simulink model "basis2"  (Simulink 6.6)
settings: Solver=ode45  StartTime=0.0  StopTime=5000  RelTol=1e-3
libraries: simulink x35, dspstat3 x3
settings Model: Creator=Paul.Dourbal  LastModifiedBy=Paul.Dourbal

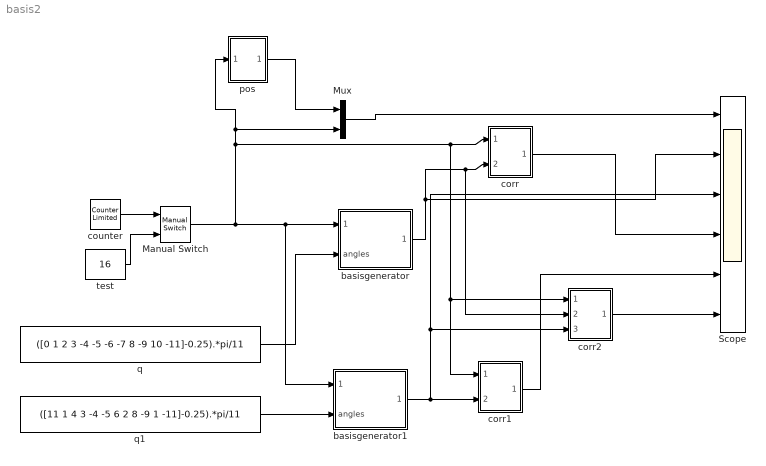
== system basis2 ==
  Manual Switch : simulink/Signal Routing/Manual Switch  SystemSampleTime=-1  sw=1  action=0  varsize=off
  Mux : Mux  Inputs=2
  Scope : Scope  NumInputPorts=6
      settings: TimeRange=64  YMin=-0.15~0~-1~-5~-5~-5  YMax=0.4~65~10~5~5~5
  basisgenerator : Subsystem
  basisgenerator1 : Subsystem
  corr : Subsystem
  corr1 : Subsystem
  corr2 : Subsystem
  counter : simulink/Sources/Counter Limited  SystemSampleTime=-1  uplimit=2^(3+3)-1  tsamp=1
  pos : Subsystem
  q : Constant  Value=([0 1 2 3 -4 -5 -6 -7 8 -9 10 -11]-0.25).*pi/11
  q1 : Constant  Value=([11 1 4 3 -4 -5 6 2 8 -9 1 -11]-0.25).*pi/11
  test : Constant  Value=16  OutDataTypeMode=uint8
  wires:
  basisgenerator/1(samples) -> Scope/2, corr/2(In2), corr2/2(sig1)
  test/1 -> Manual Switch/2
  counter/1 -> Manual Switch/1
  Manual Switch/1 -> pos/1(In1), Mux/2, corr/1(In1), corr1/1(In1), corr2/1(index), basisgenerator/1(counter), basisgenerator1/1(counter)
  pos/1(Out1) -> Mux/1
  Mux/1 -> Scope/1
  q1/1 -> basisgenerator1/2(angles)
  q/1 -> basisgenerator/2(angles)
  basisgenerator1/1(samples) -> corr1/2(In2), Scope/3, corr2/3(sig2)
  corr/1(Out1) -> Scope/4
  corr1/1(Out1) -> Scope/5
  corr2/1(Out1) -> Scope/6

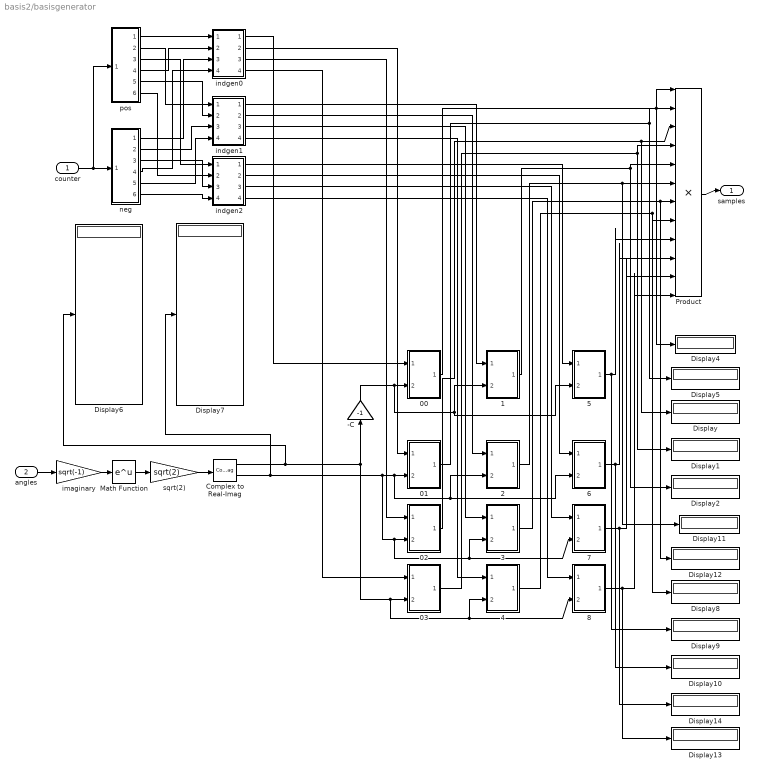
== system basis2/basisgenerator ==
  counter : Inport
  angles : Inport  Port=2
  -C : Gain  Orientation=up  Gain=-1
  00 : Subsystem
  01 : Subsystem
  02 : Subsystem
  03 : Subsystem
  1 : Subsystem
  2 : Subsystem
  3 : Subsystem
  4 : Subsystem
  5 : Subsystem
  6 : Subsystem
  7 : Subsystem
  8 : Subsystem
  Complex to Real-Imag : ComplexToRealImag
  Display{,1..2,4..14} (14 alike) : Display
  Math Function : Math  OutputSignalType=complex  SaturateOnIntegerOverflow=on
  Product : Product  Inputs=12  RndMeth=Zero
  imaginary : Gain  Gain=sqrt(-1)
  indgen0 : Subsystem
  indgen1 : Subsystem
  indgen2 : Subsystem
  neg : Subsystem
  pos : Subsystem
  sqrt(2) : Gain  Gain=sqrt(2)
  samples : Outport
  wires:
  8/1(Out1) -> Product/12, Display13/1
  7/1(Out1) -> Product/11, Display14/1
  6/1(Out1) -> Product/10, Display10/1
  5/1(Out1) -> Product/9, Display9/1
  4/1(Out1) -> Product/8, Display8/1
  3/1(Out1) -> Product/7, Display12/1
  2/1(Out1) -> Product/6, Display11/1
  1/1(Out1) -> Product/5, Display2/1
  03/1(Out1) -> Product/4, Display1/1
  02/1(Out1) -> Product/3, Display/1
  01/1(Out1) -> Product/2, Display5/1
  00/1(Out1) -> Product/1, Display4/1
  indgen2/4(Out4) -> 8/1(In1)
  indgen2/3(Out3) -> 7/1(In1)
  indgen2/2(Out2) -> 6/1(In1)
  indgen2/1(Out1) -> 5/1(In1)
  indgen1/4(Out4) -> 4/1(In1)
  indgen1/3(Out3) -> 3/1(In1)
  indgen1/2(Out2) -> 2/1(In1)
  indgen1/1(Out1) -> 1/1(In1)
  indgen0/4(Out4) -> 03/1(In1)
  indgen0/3(Out3) -> 02/1(In1)
  indgen0/2(Out2) -> 01/1(In1)
  indgen0/1(Out1) -> 00/1(In1)
  -C/1 -> 00/2(In2), 1/2(In2), 5/2(In2)
  neg/6(Out6) -> indgen2/4(In4)
  neg/3(Out3) -> indgen2/3(In3)
  pos/6(Out6) -> indgen2/2(In2)
  pos/3(Out3) -> indgen2/1(In1)
  neg/5(Out5) -> indgen1/4(In4)
  neg/2(Out2) -> indgen1/3(In3)
  pos/5(Out5) -> indgen1/2(In2)
  pos/2(Out2) -> indgen1/1(In1)
  neg/4(Out4) -> indgen0/4(In4)
  neg/1(Out1) -> indgen0/3(In3)
  pos/4(Out4) -> indgen0/2(In2)
  pos/1(Out1) -> indgen0/1(In1)
  Complex to Real-Imag/2 -> 01/2(In2), 2/2(In2), 6/2(In2), 02/2(In2), 3/2(In2), 7/2(In2), Display7/1
  Complex to Real-Imag/1 -> -C/1, 03/2(In2), 4/2(In2), 8/2(In2), Display6/1
  sqrt(2)/1 -> Complex to Real-Imag/1
  Math Function/1 -> sqrt(2)/1
  imaginary/1 -> Math Function/1
  counter/1 -> neg/1(In1), pos/1(In1)
  Product/1 -> samples/1
  angles/1 -> imaginary/1

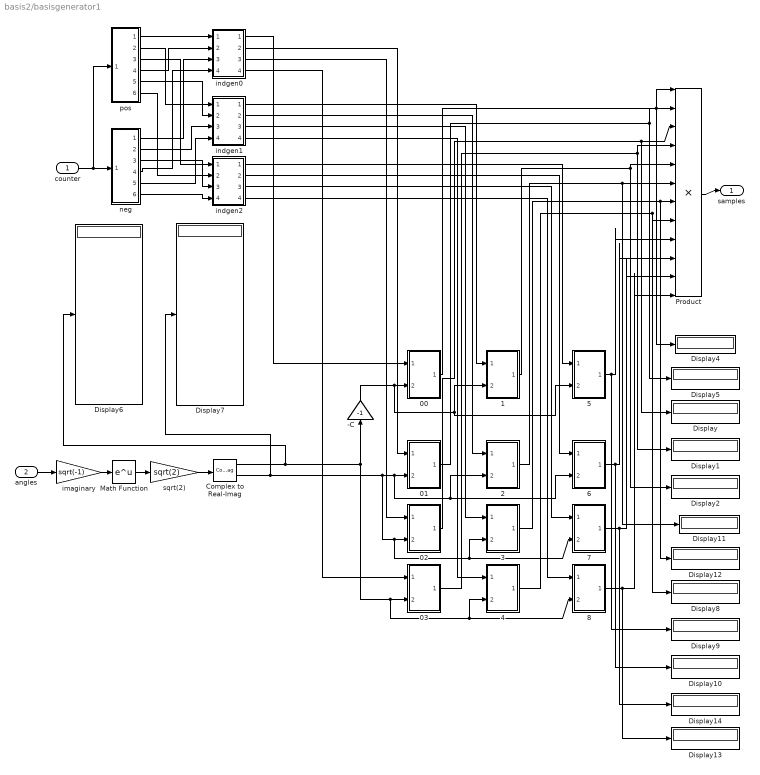
== system basis2/basisgenerator1 ==
  counter : Inport
  angles : Inport  Port=2
  -C : Gain  Orientation=up  Gain=-1
  00 : Subsystem
  01 : Subsystem
  02 : Subsystem
  03 : Subsystem
  1 : Subsystem
  2 : Subsystem
  3 : Subsystem
  4 : Subsystem
  5 : Subsystem
  6 : Subsystem
  7 : Subsystem
  8 : Subsystem
  Complex to Real-Imag : ComplexToRealImag
  Display{,1..2,4..14} (14 alike) : Display
  Math Function : Math  OutputSignalType=complex  SaturateOnIntegerOverflow=on
  Product : Product  Inputs=12  RndMeth=Zero
  imaginary : Gain  Gain=sqrt(-1)
  indgen0 : Subsystem
  indgen1 : Subsystem
  indgen2 : Subsystem
  neg : Subsystem
  pos : Subsystem
  sqrt(2) : Gain  Gain=sqrt(2)
  samples : Outport
  wires:
  8/1(Out1) -> Product/12, Display13/1
  7/1(Out1) -> Product/11, Display14/1
  6/1(Out1) -> Product/10, Display10/1
  5/1(Out1) -> Product/9, Display9/1
  4/1(Out1) -> Product/8, Display8/1
  3/1(Out1) -> Product/7, Display12/1
  2/1(Out1) -> Product/6, Display11/1
  1/1(Out1) -> Product/5, Display2/1
  03/1(Out1) -> Product/4, Display1/1
  02/1(Out1) -> Product/3, Display/1
  01/1(Out1) -> Product/2, Display5/1
  00/1(Out1) -> Product/1, Display4/1
  indgen2/4(Out4) -> 8/1(In1)
  indgen2/3(Out3) -> 7/1(In1)
  indgen2/2(Out2) -> 6/1(In1)
  indgen2/1(Out1) -> 5/1(In1)
  indgen1/4(Out4) -> 4/1(In1)
  indgen1/3(Out3) -> 3/1(In1)
  indgen1/2(Out2) -> 2/1(In1)
  indgen1/1(Out1) -> 1/1(In1)
  indgen0/4(Out4) -> 03/1(In1)
  indgen0/3(Out3) -> 02/1(In1)
  indgen0/2(Out2) -> 01/1(In1)
  indgen0/1(Out1) -> 00/1(In1)
  -C/1 -> 00/2(In2), 1/2(In2), 5/2(In2)
  neg/6(Out6) -> indgen2/4(In4)
  neg/3(Out3) -> indgen2/3(In3)
  pos/6(Out6) -> indgen2/2(In2)
  pos/3(Out3) -> indgen2/1(In1)
  neg/5(Out5) -> indgen1/4(In4)
  neg/2(Out2) -> indgen1/3(In3)
  pos/5(Out5) -> indgen1/2(In2)
  pos/2(Out2) -> indgen1/1(In1)
  neg/4(Out4) -> indgen0/4(In4)
  neg/1(Out1) -> indgen0/3(In3)
  pos/4(Out4) -> indgen0/2(In2)
  pos/1(Out1) -> indgen0/1(In1)
  Complex to Real-Imag/2 -> 01/2(In2), 2/2(In2), 6/2(In2), 02/2(In2), 3/2(In2), 7/2(In2), Display7/1
  Complex to Real-Imag/1 -> -C/1, 03/2(In2), 4/2(In2), 8/2(In2), Display6/1
  sqrt(2)/1 -> Complex to Real-Imag/1
  Math Function/1 -> sqrt(2)/1
  imaginary/1 -> Math Function/1
  counter/1 -> neg/1(In1), pos/1(In1)
  Product/1 -> samples/1
  angles/1 -> imaginary/1

== system basis2/corr ==
  In1 : Inport
  In2 : Inport  Port=2
  Autocorrelation : dspstat3/Autocorrelation  DialogController=dspDDGCreate  DialogControllerArgs=DataTag0  AllPositiveLags=on  maxlag=36  bias=None  domain=Time  roundingMode=Floor  overflowMode=off
  Tapped Delay : simulink/Discrete/Tapped Delay  vinit=0.0  samptime=1/64  NumDelays=64  DelayOrder=Oldest  includeCurrent=off
  mux : Subsystem
  Out1 : Outport
  wires:
  Tapped Delay/1 -> Autocorrelation/1
  Autocorrelation/1 -> mux/2(In2)
  In1/1 -> mux/1(In1)
  In2/1 -> Tapped Delay/1
  mux/1(Out1) -> Out1/1

== system basis2/corr1 ==
  In1 : Inport
  In2 : Inport  Port=2
  Autocorrelation : dspstat3/Autocorrelation  DialogController=dspDDGCreate  DialogControllerArgs=DataTag1  AllPositiveLags=on  maxlag=36  bias=None  domain=Time  roundingMode=Floor  overflowMode=off
  Tapped Delay : simulink/Discrete/Tapped Delay  vinit=0.0  samptime=1/64  NumDelays=64  DelayOrder=Oldest  includeCurrent=off
  mux : Subsystem
  Out1 : Outport
  wires:
  Tapped Delay/1 -> Autocorrelation/1
  Autocorrelation/1 -> mux/2(In2)
  In1/1 -> mux/1(In1)
  In2/1 -> Tapped Delay/1
  mux/1(Out1) -> Out1/1

== system basis2/corr2 ==
  index : Inport
  sig1 : Inport  Port=2
  sig2 : Inport  Port=3
  Correlation : dspstat3/Correlation  DialogController=dspDDGCreate  DialogControllerArgs=DataTag2  domain=Time  roundingMode=Floor  overflowMode=off
  Tapped Delay : simulink/Discrete/Tapped Delay  vinit=0.0  samptime=1/64  NumDelays=64  DelayOrder=Oldest  includeCurrent=off
  Tapped Delay1 : simulink/Discrete/Tapped Delay  vinit=0.0  samptime=1/64  NumDelays=64  DelayOrder=Oldest  includeCurrent=off
  mux : Subsystem
  Out1 : Outport
  wires:
  Tapped Delay/1 -> Correlation/1
  Correlation/1 -> mux/2(In2)
  index/1 -> mux/1(In1)
  sig1/1 -> Tapped Delay/1
  mux/1(Out1) -> Out1/1
  sig2/1 -> Tapped Delay1/1
  Tapped Delay1/1 -> Correlation/2

== system basis2/pos ==
  In1 : Inport  Orientation=up
  Extract Bits3 : simulink/Logic and Bit Operations/Extract Bits  SystemSampleTime=-1  bitsToExtract=Range of bits  numBits=8  bitIdxRange=[2 2]  outScalingMode=Treat bit field as an integer
  Extract Bits4 : simulink/Logic and Bit Operations/Extract Bits  SystemSampleTime=-1  bitsToExtract=Range of bits  numBits=8  bitIdxRange=[1 1]  outScalingMode=Treat bit field as an integer
  Extract Bits5 : simulink/Logic and Bit Operations/Extract Bits  SystemSampleTime=-1  bitsToExtract=Range of bits  numBits=8  bitIdxRange=[0 0]  outScalingMode=Treat bit field as an integer
  ws : Subsystem
  Out1 : Outport
  wires:
  Extract Bits5/1 -> ws/1(in0)
  In1/1 -> Extract Bits3/1, Extract Bits5/1, Extract Bits4/1
  Extract Bits4/1 -> ws/2(in1)
  Extract Bits3/1 -> ws/3(in2)
  ws/1(Out1) -> Out1/1

== system basis2/basisgenerator/00 ==
  In1 : Inport
  In2 : Inport  Port=2
  C : MultiPortSwitch  Inputs=12  zeroidx=on
  Demux3 : Demux  Outputs=12
  Out1 : Outport
  wires:
  Demux3/1 -> C/2
  Demux3/2 -> C/3
  Demux3/3 -> C/4
  Demux3/4 -> C/5
  Demux3/5 -> C/6
  Demux3/6 -> C/7
  Demux3/7 -> C/8
  Demux3/8 -> C/9
  Demux3/9 -> C/10
  Demux3/10 -> C/11
  Demux3/11 -> C/12
  Demux3/12 -> C/13
  In1/1 -> C/1
  C/1 -> Out1/1
  In2/1 -> Demux3/1

== system basis2/basisgenerator/01 ==
  In1 : Inport
  In2 : Inport  Port=2
  C : MultiPortSwitch  Inputs=12  zeroidx=on
  Demux3 : Demux  Outputs=12
  Out1 : Outport
  wires:
  Demux3/1 -> C/2
  Demux3/2 -> C/3
  Demux3/3 -> C/4
  Demux3/4 -> C/5
  Demux3/5 -> C/6
  Demux3/6 -> C/7
  Demux3/7 -> C/8
  Demux3/8 -> C/9
  Demux3/9 -> C/10
  Demux3/10 -> C/11
  Demux3/11 -> C/12
  Demux3/12 -> C/13
  In1/1 -> C/1
  C/1 -> Out1/1
  In2/1 -> Demux3/1

== system basis2/basisgenerator/02 ==
  In1 : Inport
  In2 : Inport  Port=2
  C : MultiPortSwitch  Inputs=12  zeroidx=on
  Demux3 : Demux  Outputs=12
  Out1 : Outport
  wires:
  Demux3/1 -> C/2
  Demux3/2 -> C/3
  Demux3/3 -> C/4
  Demux3/4 -> C/5
  Demux3/5 -> C/6
  Demux3/6 -> C/7
  Demux3/7 -> C/8
  Demux3/8 -> C/9
  Demux3/9 -> C/10
  Demux3/10 -> C/11
  Demux3/11 -> C/12
  Demux3/12 -> C/13
  In1/1 -> C/1
  C/1 -> Out1/1
  In2/1 -> Demux3/1

== system basis2/basisgenerator/03 ==
  In1 : Inport
  In2 : Inport  Port=2
  C : MultiPortSwitch  Inputs=12  zeroidx=on
  Demux3 : Demux  Outputs=12
  Out1 : Outport
  wires:
  Demux3/1 -> C/2
  Demux3/2 -> C/3
  Demux3/3 -> C/4
  Demux3/4 -> C/5
  Demux3/5 -> C/6
  Demux3/6 -> C/7
  Demux3/7 -> C/8
  Demux3/8 -> C/9
  Demux3/9 -> C/10
  Demux3/10 -> C/11
  Demux3/11 -> C/12
  Demux3/12 -> C/13
  In1/1 -> C/1
  C/1 -> Out1/1
  In2/1 -> Demux3/1

== system basis2/basisgenerator/1 ==
  In1 : Inport
  In2 : Inport  Port=2
  C : MultiPortSwitch  Inputs=12  zeroidx=on
  Demux3 : Demux  Outputs=12
  Out1 : Outport
  wires:
  Demux3/1 -> C/2
  Demux3/2 -> C/3
  Demux3/3 -> C/4
  Demux3/4 -> C/5
  Demux3/5 -> C/6
  Demux3/6 -> C/7
  Demux3/7 -> C/8
  Demux3/8 -> C/9
  Demux3/9 -> C/10
  Demux3/10 -> C/11
  Demux3/11 -> C/12
  Demux3/12 -> C/13
  In1/1 -> C/1
  C/1 -> Out1/1
  In2/1 -> Demux3/1

== system basis2/basisgenerator/2 ==
  In1 : Inport
  In2 : Inport  Port=2
  C : MultiPortSwitch  Inputs=12  zeroidx=on
  Demux3 : Demux  Outputs=12
  Out1 : Outport
  wires:
  Demux3/1 -> C/2
  Demux3/2 -> C/3
  Demux3/3 -> C/4
  Demux3/4 -> C/5
  Demux3/5 -> C/6
  Demux3/6 -> C/7
  Demux3/7 -> C/8
  Demux3/8 -> C/9
  Demux3/9 -> C/10
  Demux3/10 -> C/11
  Demux3/11 -> C/12
  Demux3/12 -> C/13
  In1/1 -> C/1
  C/1 -> Out1/1
  In2/1 -> Demux3/1

== system basis2/basisgenerator/3 ==
  In1 : Inport
  In2 : Inport  Port=2
  C : MultiPortSwitch  Inputs=12  zeroidx=on
  Demux3 : Demux  Outputs=12
  Out1 : Outport
  wires:
  Demux3/1 -> C/2
  Demux3/2 -> C/3
  Demux3/3 -> C/4
  Demux3/4 -> C/5
  Demux3/5 -> C/6
  Demux3/6 -> C/7
  Demux3/7 -> C/8
  Demux3/8 -> C/9
  Demux3/9 -> C/10
  Demux3/10 -> C/11
  Demux3/11 -> C/12
  Demux3/12 -> C/13
  In1/1 -> C/1
  C/1 -> Out1/1
  In2/1 -> Demux3/1

== system basis2/basisgenerator/4 ==
  In1 : Inport
  In2 : Inport  Port=2
  C : MultiPortSwitch  Inputs=12  zeroidx=on
  Demux3 : Demux  Outputs=12
  Out1 : Outport
  wires:
  Demux3/1 -> C/2
  Demux3/2 -> C/3
  Demux3/3 -> C/4
  Demux3/4 -> C/5
  Demux3/5 -> C/6
  Demux3/6 -> C/7
  Demux3/7 -> C/8
  Demux3/8 -> C/9
  Demux3/9 -> C/10
  Demux3/10 -> C/11
  Demux3/11 -> C/12
  Demux3/12 -> C/13
  In1/1 -> C/1
  C/1 -> Out1/1
  In2/1 -> Demux3/1

== system basis2/basisgenerator/5 ==
  In1 : Inport
  In2 : Inport  Port=2
  C : MultiPortSwitch  Inputs=12  zeroidx=on
  Demux3 : Demux  Outputs=12
  Out1 : Outport
  wires:
  Demux3/1 -> C/2
  Demux3/2 -> C/3
  Demux3/3 -> C/4
  Demux3/4 -> C/5
  Demux3/5 -> C/6
  Demux3/6 -> C/7
  Demux3/7 -> C/8
  Demux3/8 -> C/9
  Demux3/9 -> C/10
  Demux3/10 -> C/11
  Demux3/11 -> C/12
  Demux3/12 -> C/13
  In1/1 -> C/1
  C/1 -> Out1/1
  In2/1 -> Demux3/1

== system basis2/basisgenerator/6 ==
  In1 : Inport
  In2 : Inport  Port=2
  C : MultiPortSwitch  Inputs=12  zeroidx=on
  Demux3 : Demux  Outputs=12
  Out1 : Outport
  wires:
  Demux3/1 -> C/2
  Demux3/2 -> C/3
  Demux3/3 -> C/4
  Demux3/4 -> C/5
  Demux3/5 -> C/6
  Demux3/6 -> C/7
  Demux3/7 -> C/8
  Demux3/8 -> C/9
  Demux3/9 -> C/10
  Demux3/10 -> C/11
  Demux3/11 -> C/12
  Demux3/12 -> C/13
  In1/1 -> C/1
  C/1 -> Out1/1
  In2/1 -> Demux3/1

== system basis2/basisgenerator/7 ==
  In1 : Inport
  In2 : Inport  Port=2
  C : MultiPortSwitch  Inputs=12  zeroidx=on
  Demux3 : Demux  Outputs=12
  Out1 : Outport
  wires:
  Demux3/1 -> C/2
  Demux3/2 -> C/3
  Demux3/3 -> C/4
  Demux3/4 -> C/5
  Demux3/5 -> C/6
  Demux3/6 -> C/7
  Demux3/7 -> C/8
  Demux3/8 -> C/9
  Demux3/9 -> C/10
  Demux3/10 -> C/11
  Demux3/11 -> C/12
  Demux3/12 -> C/13
  In1/1 -> C/1
  C/1 -> Out1/1
  In2/1 -> Demux3/1

== system basis2/basisgenerator/8 ==
  In1 : Inport
  In2 : Inport  Port=2
  C : MultiPortSwitch  Inputs=12  zeroidx=on
  Demux3 : Demux  Outputs=12
  Out1 : Outport
  wires:
  Demux3/1 -> C/2
  Demux3/2 -> C/3
  Demux3/3 -> C/4
  Demux3/4 -> C/5
  Demux3/5 -> C/6
  Demux3/6 -> C/7
  Demux3/7 -> C/8
  Demux3/8 -> C/9
  Demux3/9 -> C/10
  Demux3/10 -> C/11
  Demux3/11 -> C/12
  Demux3/12 -> C/13
  In1/1 -> C/1
  C/1 -> Out1/1
  In2/1 -> Demux3/1

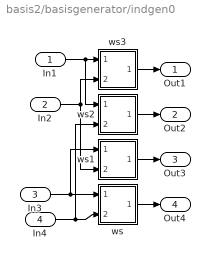
== system basis2/basisgenerator/indgen0 ==
  In1 : Inport
  In2 : Inport  Port=2
  In3 : Inport  Port=3
  In4 : Inport  Port=4
  ws : Subsystem
  ws1 : Subsystem
  ws2 : Subsystem
  ws3 : Subsystem
  Out1 : Outport
  Out2 : Outport  Port=2
  Out3 : Outport  Port=3
  Out4 : Outport  Port=4
  wires:
  In3/1 -> ws1/1(In1), ws/1(In1)
  In4/1 -> ws2/2(In2), ws/2(In2)
  In2/1 -> ws3/2(In2), ws1/2(In2)
  In1/1 -> ws3/1(In1), ws2/1(In1)
  ws3/1(Out1) -> Out1/1
  ws2/1(Out1) -> Out2/1
  ws1/1(Out1) -> Out3/1
  ws/1(Out1) -> Out4/1

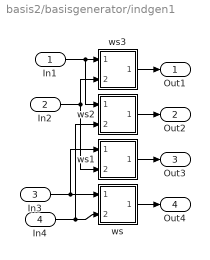
== system basis2/basisgenerator/indgen1 ==
  In1 : Inport
  In2 : Inport  Port=2
  In3 : Inport  Port=3
  In4 : Inport  Port=4
  ws : Subsystem
  ws1 : Subsystem
  ws2 : Subsystem
  ws3 : Subsystem
  Out1 : Outport
  Out2 : Outport  Port=2
  Out3 : Outport  Port=3
  Out4 : Outport  Port=4
  wires:
  In3/1 -> ws1/1(In1), ws/1(In1)
  In4/1 -> ws2/2(In2), ws/2(In2)
  In2/1 -> ws3/2(In2), ws1/2(In2)
  In1/1 -> ws3/1(In1), ws2/1(In1)
  ws3/1(Out1) -> Out1/1
  ws2/1(Out1) -> Out2/1
  ws1/1(Out1) -> Out3/1
  ws/1(Out1) -> Out4/1

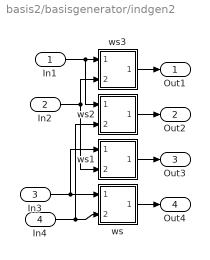
== system basis2/basisgenerator/indgen2 ==
  In1 : Inport
  In2 : Inport  Port=2
  In3 : Inport  Port=3
  In4 : Inport  Port=4
  ws : Subsystem
  ws1 : Subsystem
  ws2 : Subsystem
  ws3 : Subsystem
  Out1 : Outport
  Out2 : Outport  Port=2
  Out3 : Outport  Port=3
  Out4 : Outport  Port=4
  wires:
  In3/1 -> ws1/1(In1), ws/1(In1)
  In4/1 -> ws2/2(In2), ws/2(In2)
  In2/1 -> ws3/2(In2), ws1/2(In2)
  In1/1 -> ws3/1(In1), ws2/1(In1)
  ws3/1(Out1) -> Out1/1
  ws2/1(Out1) -> Out2/1
  ws1/1(Out1) -> Out3/1
  ws/1(Out1) -> Out4/1

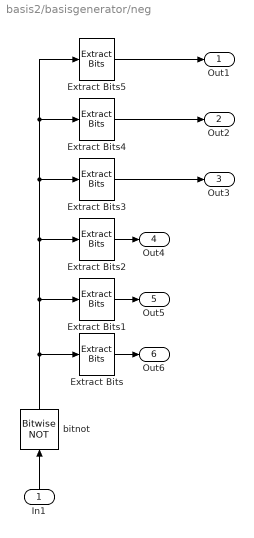
== system basis2/basisgenerator/neg ==
  In1 : Inport  Orientation=up
  Extract Bits : simulink/Logic and Bit Operations/Extract Bits  SystemSampleTime=-1  bitsToExtract=Range of bits  numBits=8  bitIdxRange=[5 5]  outScalingMode=Treat bit field as an integer
  Extract Bits1 : simulink/Logic and Bit Operations/Extract Bits  SystemSampleTime=-1  bitsToExtract=Range of bits  numBits=8  bitIdxRange=[4 4]  outScalingMode=Treat bit field as an integer
  Extract Bits2 : simulink/Logic and Bit Operations/Extract Bits  SystemSampleTime=-1  bitsToExtract=Range of bits  numBits=8  bitIdxRange=[3 3]  outScalingMode=Treat bit field as an integer
  Extract Bits3 : simulink/Logic and Bit Operations/Extract Bits  SystemSampleTime=-1  bitsToExtract=Range of bits  numBits=8  bitIdxRange=[2 2]  outScalingMode=Treat bit field as an integer
  Extract Bits4 : simulink/Logic and Bit Operations/Extract Bits  SystemSampleTime=-1  bitsToExtract=Range of bits  numBits=8  bitIdxRange=[1 1]  outScalingMode=Treat bit field as an integer
  Extract Bits5 : simulink/Logic and Bit Operations/Extract Bits  SystemSampleTime=-1  bitsToExtract=Range of bits  numBits=8  bitIdxRange=[0 0]  outScalingMode=Treat bit field as an integer
  bitnot : simulink/Logic and Bit Operations/Bitwise Operator  Orientation=up  logicop=NOT  UseBitMask=off  BitMask=bin2dec('11011001')  BitMaskRealWorld=Stored Integer
  Out1 : Outport
  Out2 : Outport  Port=2
  Out3 : Outport  Port=3
  Out4 : Outport  Port=4
  Out5 : Outport  Port=5
  Out6 : Outport  Port=6
  wires:
  Extract Bits5/1 -> Out1/1
  Extract Bits4/1 -> Out2/1
  Extract Bits3/1 -> Out3/1
  Extract Bits2/1 -> Out4/1
  In1/1 -> bitnot/1
  Extract Bits1/1 -> Out5/1
  Extract Bits/1 -> Out6/1
  bitnot/1 -> Extract Bits1/1, Extract Bits2/1, Extract Bits3/1, Extract Bits5/1, Extract Bits4/1, Extract Bits/1

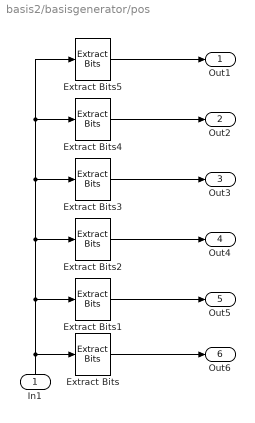
== system basis2/basisgenerator/pos ==
  In1 : Inport  Orientation=up
  Extract Bits : simulink/Logic and Bit Operations/Extract Bits  SystemSampleTime=-1  bitsToExtract=Range of bits  numBits=8  bitIdxRange=[5 5]  outScalingMode=Treat bit field as an integer
  Extract Bits1 : simulink/Logic and Bit Operations/Extract Bits  SystemSampleTime=-1  bitsToExtract=Range of bits  numBits=8  bitIdxRange=[4 4]  outScalingMode=Treat bit field as an integer
  Extract Bits2 : simulink/Logic and Bit Operations/Extract Bits  SystemSampleTime=-1  bitsToExtract=Range of bits  numBits=8  bitIdxRange=[3 3]  outScalingMode=Treat bit field as an integer
  Extract Bits3 : simulink/Logic and Bit Operations/Extract Bits  SystemSampleTime=-1  bitsToExtract=Range of bits  numBits=8  bitIdxRange=[2 2]  outScalingMode=Treat bit field as an integer
  Extract Bits4 : simulink/Logic and Bit Operations/Extract Bits  SystemSampleTime=-1  bitsToExtract=Range of bits  numBits=8  bitIdxRange=[1 1]  outScalingMode=Treat bit field as an integer
  Extract Bits5 : simulink/Logic and Bit Operations/Extract Bits  SystemSampleTime=-1  bitsToExtract=Range of bits  numBits=8  bitIdxRange=[0 0]  outScalingMode=Treat bit field as an integer
  Out1 : Outport
  Out2 : Outport  Port=2
  Out3 : Outport  Port=3
  Out4 : Outport  Port=4
  Out5 : Outport  Port=5
  Out6 : Outport  Port=6
  wires:
  Extract Bits5/1 -> Out1/1
  Extract Bits4/1 -> Out2/1
  Extract Bits3/1 -> Out3/1
  Extract Bits2/1 -> Out4/1
  In1/1 -> Extract Bits1/1, Extract Bits2/1, Extract Bits3/1, Extract Bits5/1, Extract Bits4/1, Extract Bits/1
  Extract Bits1/1 -> Out5/1
  Extract Bits/1 -> Out6/1

== system basis2/basisgenerator1/00 ==
  In1 : Inport
  In2 : Inport  Port=2
  C : MultiPortSwitch  Inputs=12  zeroidx=on
  Demux3 : Demux  Outputs=12
  Out1 : Outport
  wires:
  Demux3/1 -> C/2
  Demux3/2 -> C/3
  Demux3/3 -> C/4
  Demux3/4 -> C/5
  Demux3/5 -> C/6
  Demux3/6 -> C/7
  Demux3/7 -> C/8
  Demux3/8 -> C/9
  Demux3/9 -> C/10
  Demux3/10 -> C/11
  Demux3/11 -> C/12
  Demux3/12 -> C/13
  In1/1 -> C/1
  C/1 -> Out1/1
  In2/1 -> Demux3/1

== system basis2/basisgenerator1/01 ==
  In1 : Inport
  In2 : Inport  Port=2
  C : MultiPortSwitch  Inputs=12  zeroidx=on
  Demux3 : Demux  Outputs=12
  Out1 : Outport
  wires:
  Demux3/1 -> C/2
  Demux3/2 -> C/3
  Demux3/3 -> C/4
  Demux3/4 -> C/5
  Demux3/5 -> C/6
  Demux3/6 -> C/7
  Demux3/7 -> C/8
  Demux3/8 -> C/9
  Demux3/9 -> C/10
  Demux3/10 -> C/11
  Demux3/11 -> C/12
  Demux3/12 -> C/13
  In1/1 -> C/1
  C/1 -> Out1/1
  In2/1 -> Demux3/1

== system basis2/basisgenerator1/02 ==
  In1 : Inport
  In2 : Inport  Port=2
  C : MultiPortSwitch  Inputs=12  zeroidx=on
  Demux3 : Demux  Outputs=12
  Out1 : Outport
  wires:
  Demux3/1 -> C/2
  Demux3/2 -> C/3
  Demux3/3 -> C/4
  Demux3/4 -> C/5
  Demux3/5 -> C/6
  Demux3/6 -> C/7
  Demux3/7 -> C/8
  Demux3/8 -> C/9
  Demux3/9 -> C/10
  Demux3/10 -> C/11
  Demux3/11 -> C/12
  Demux3/12 -> C/13
  In1/1 -> C/1
  C/1 -> Out1/1
  In2/1 -> Demux3/1

== system basis2/basisgenerator1/03 ==
  In1 : Inport
  In2 : Inport  Port=2
  C : MultiPortSwitch  Inputs=12  zeroidx=on
  Demux3 : Demux  Outputs=12
  Out1 : Outport
  wires:
  Demux3/1 -> C/2
  Demux3/2 -> C/3
  Demux3/3 -> C/4
  Demux3/4 -> C/5
  Demux3/5 -> C/6
  Demux3/6 -> C/7
  Demux3/7 -> C/8
  Demux3/8 -> C/9
  Demux3/9 -> C/10
  Demux3/10 -> C/11
  Demux3/11 -> C/12
  Demux3/12 -> C/13
  In1/1 -> C/1
  C/1 -> Out1/1
  In2/1 -> Demux3/1

== system basis2/basisgenerator1/1 ==
  In1 : Inport
  In2 : Inport  Port=2
  C : MultiPortSwitch  Inputs=12  zeroidx=on
  Demux3 : Demux  Outputs=12
  Out1 : Outport
  wires:
  Demux3/1 -> C/2
  Demux3/2 -> C/3
  Demux3/3 -> C/4
  Demux3/4 -> C/5
  Demux3/5 -> C/6
  Demux3/6 -> C/7
  Demux3/7 -> C/8
  Demux3/8 -> C/9
  Demux3/9 -> C/10
  Demux3/10 -> C/11
  Demux3/11 -> C/12
  Demux3/12 -> C/13
  In1/1 -> C/1
  C/1 -> Out1/1
  In2/1 -> Demux3/1

== system basis2/basisgenerator1/2 ==
  In1 : Inport
  In2 : Inport  Port=2
  C : MultiPortSwitch  Inputs=12  zeroidx=on
  Demux3 : Demux  Outputs=12
  Out1 : Outport
  wires:
  Demux3/1 -> C/2
  Demux3/2 -> C/3
  Demux3/3 -> C/4
  Demux3/4 -> C/5
  Demux3/5 -> C/6
  Demux3/6 -> C/7
  Demux3/7 -> C/8
  Demux3/8 -> C/9
  Demux3/9 -> C/10
  Demux3/10 -> C/11
  Demux3/11 -> C/12
  Demux3/12 -> C/13
  In1/1 -> C/1
  C/1 -> Out1/1
  In2/1 -> Demux3/1

== system basis2/basisgenerator1/3 ==
  In1 : Inport
  In2 : Inport  Port=2
  C : MultiPortSwitch  Inputs=12  zeroidx=on
  Demux3 : Demux  Outputs=12
  Out1 : Outport
  wires:
  Demux3/1 -> C/2
  Demux3/2 -> C/3
  Demux3/3 -> C/4
  Demux3/4 -> C/5
  Demux3/5 -> C/6
  Demux3/6 -> C/7
  Demux3/7 -> C/8
  Demux3/8 -> C/9
  Demux3/9 -> C/10
  Demux3/10 -> C/11
  Demux3/11 -> C/12
  Demux3/12 -> C/13
  In1/1 -> C/1
  C/1 -> Out1/1
  In2/1 -> Demux3/1

== system basis2/basisgenerator1/4 ==
  In1 : Inport
  In2 : Inport  Port=2
  C : MultiPortSwitch  Inputs=12  zeroidx=on
  Demux3 : Demux  Outputs=12
  Out1 : Outport
  wires:
  Demux3/1 -> C/2
  Demux3/2 -> C/3
  Demux3/3 -> C/4
  Demux3/4 -> C/5
  Demux3/5 -> C/6
  Demux3/6 -> C/7
  Demux3/7 -> C/8
  Demux3/8 -> C/9
  Demux3/9 -> C/10
  Demux3/10 -> C/11
  Demux3/11 -> C/12
  Demux3/12 -> C/13
  In1/1 -> C/1
  C/1 -> Out1/1
  In2/1 -> Demux3/1

== system basis2/basisgenerator1/5 ==
  In1 : Inport
  In2 : Inport  Port=2
  C : MultiPortSwitch  Inputs=12  zeroidx=on
  Demux3 : Demux  Outputs=12
  Out1 : Outport
  wires:
  Demux3/1 -> C/2
  Demux3/2 -> C/3
  Demux3/3 -> C/4
  Demux3/4 -> C/5
  Demux3/5 -> C/6
  Demux3/6 -> C/7
  Demux3/7 -> C/8
  Demux3/8 -> C/9
  Demux3/9 -> C/10
  Demux3/10 -> C/11
  Demux3/11 -> C/12
  Demux3/12 -> C/13
  In1/1 -> C/1
  C/1 -> Out1/1
  In2/1 -> Demux3/1

== system basis2/basisgenerator1/6 ==
  In1 : Inport
  In2 : Inport  Port=2
  C : MultiPortSwitch  Inputs=12  zeroidx=on
  Demux3 : Demux  Outputs=12
  Out1 : Outport
  wires:
  Demux3/1 -> C/2
  Demux3/2 -> C/3
  Demux3/3 -> C/4
  Demux3/4 -> C/5
  Demux3/5 -> C/6
  Demux3/6 -> C/7
  Demux3/7 -> C/8
  Demux3/8 -> C/9
  Demux3/9 -> C/10
  Demux3/10 -> C/11
  Demux3/11 -> C/12
  Demux3/12 -> C/13
  In1/1 -> C/1
  C/1 -> Out1/1
  In2/1 -> Demux3/1

== system basis2/basisgenerator1/7 ==
  In1 : Inport
  In2 : Inport  Port=2
  C : MultiPortSwitch  Inputs=12  zeroidx=on
  Demux3 : Demux  Outputs=12
  Out1 : Outport
  wires:
  Demux3/1 -> C/2
  Demux3/2 -> C/3
  Demux3/3 -> C/4
  Demux3/4 -> C/5
  Demux3/5 -> C/6
  Demux3/6 -> C/7
  Demux3/7 -> C/8
  Demux3/8 -> C/9
  Demux3/9 -> C/10
  Demux3/10 -> C/11
  Demux3/11 -> C/12
  Demux3/12 -> C/13
  In1/1 -> C/1
  C/1 -> Out1/1
  In2/1 -> Demux3/1

== system basis2/basisgenerator1/8 ==
  In1 : Inport
  In2 : Inport  Port=2
  C : MultiPortSwitch  Inputs=12  zeroidx=on
  Demux3 : Demux  Outputs=12
  Out1 : Outport
  wires:
  Demux3/1 -> C/2
  Demux3/2 -> C/3
  Demux3/3 -> C/4
  Demux3/4 -> C/5
  Demux3/5 -> C/6
  Demux3/6 -> C/7
  Demux3/7 -> C/8
  Demux3/8 -> C/9
  Demux3/9 -> C/10
  Demux3/10 -> C/11
  Demux3/11 -> C/12
  Demux3/12 -> C/13
  In1/1 -> C/1
  C/1 -> Out1/1
  In2/1 -> Demux3/1

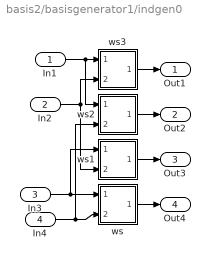
== system basis2/basisgenerator1/indgen0 ==
  In1 : Inport
  In2 : Inport  Port=2
  In3 : Inport  Port=3
  In4 : Inport  Port=4
  ws : Subsystem
  ws1 : Subsystem
  ws2 : Subsystem
  ws3 : Subsystem
  Out1 : Outport
  Out2 : Outport  Port=2
  Out3 : Outport  Port=3
  Out4 : Outport  Port=4
  wires:
  In3/1 -> ws1/1(In1), ws/1(In1)
  In4/1 -> ws2/2(In2), ws/2(In2)
  In2/1 -> ws3/2(In2), ws1/2(In2)
  In1/1 -> ws3/1(In1), ws2/1(In1)
  ws3/1(Out1) -> Out1/1
  ws2/1(Out1) -> Out2/1
  ws1/1(Out1) -> Out3/1
  ws/1(Out1) -> Out4/1

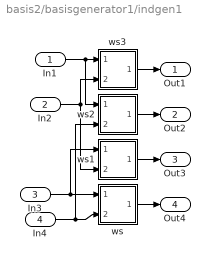
== system basis2/basisgenerator1/indgen1 ==
  In1 : Inport
  In2 : Inport  Port=2
  In3 : Inport  Port=3
  In4 : Inport  Port=4
  ws : Subsystem
  ws1 : Subsystem
  ws2 : Subsystem
  ws3 : Subsystem
  Out1 : Outport
  Out2 : Outport  Port=2
  Out3 : Outport  Port=3
  Out4 : Outport  Port=4
  wires:
  In3/1 -> ws1/1(In1), ws/1(In1)
  In4/1 -> ws2/2(In2), ws/2(In2)
  In2/1 -> ws3/2(In2), ws1/2(In2)
  In1/1 -> ws3/1(In1), ws2/1(In1)
  ws3/1(Out1) -> Out1/1
  ws2/1(Out1) -> Out2/1
  ws1/1(Out1) -> Out3/1
  ws/1(Out1) -> Out4/1

== system basis2/basisgenerator1/indgen2 ==
  In1 : Inport
  In2 : Inport  Port=2
  In3 : Inport  Port=3
  In4 : Inport  Port=4
  ws : Subsystem
  ws1 : Subsystem
  ws2 : Subsystem
  ws3 : Subsystem
  Out1 : Outport
  Out2 : Outport  Port=2
  Out3 : Outport  Port=3
  Out4 : Outport  Port=4
  wires:
  In3/1 -> ws1/1(In1), ws/1(In1)
  In4/1 -> ws2/2(In2), ws/2(In2)
  In2/1 -> ws3/2(In2), ws1/2(In2)
  In1/1 -> ws3/1(In1), ws2/1(In1)
  ws3/1(Out1) -> Out1/1
  ws2/1(Out1) -> Out2/1
  ws1/1(Out1) -> Out3/1
  ws/1(Out1) -> Out4/1

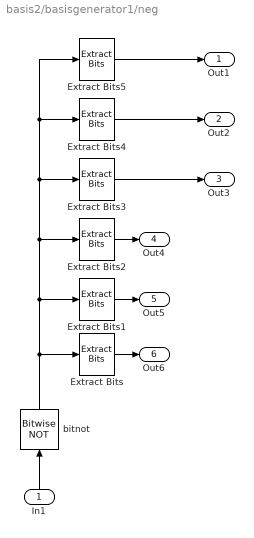
== system basis2/basisgenerator1/neg ==
  In1 : Inport  Orientation=up
  Extract Bits : simulink/Logic and Bit Operations/Extract Bits  SystemSampleTime=-1  bitsToExtract=Range of bits  numBits=8  bitIdxRange=[5 5]  outScalingMode=Treat bit field as an integer
  Extract Bits1 : simulink/Logic and Bit Operations/Extract Bits  SystemSampleTime=-1  bitsToExtract=Range of bits  numBits=8  bitIdxRange=[4 4]  outScalingMode=Treat bit field as an integer
  Extract Bits2 : simulink/Logic and Bit Operations/Extract Bits  SystemSampleTime=-1  bitsToExtract=Range of bits  numBits=8  bitIdxRange=[3 3]  outScalingMode=Treat bit field as an integer
  Extract Bits3 : simulink/Logic and Bit Operations/Extract Bits  SystemSampleTime=-1  bitsToExtract=Range of bits  numBits=8  bitIdxRange=[2 2]  outScalingMode=Treat bit field as an integer
  Extract Bits4 : simulink/Logic and Bit Operations/Extract Bits  SystemSampleTime=-1  bitsToExtract=Range of bits  numBits=8  bitIdxRange=[1 1]  outScalingMode=Treat bit field as an integer
  Extract Bits5 : simulink/Logic and Bit Operations/Extract Bits  SystemSampleTime=-1  bitsToExtract=Range of bits  numBits=8  bitIdxRange=[0 0]  outScalingMode=Treat bit field as an integer
  bitnot : simulink/Logic and Bit Operations/Bitwise Operator  Orientation=up  logicop=NOT  UseBitMask=off  BitMask=bin2dec('11011001')  BitMaskRealWorld=Stored Integer
  Out1 : Outport
  Out2 : Outport  Port=2
  Out3 : Outport  Port=3
  Out4 : Outport  Port=4
  Out5 : Outport  Port=5
  Out6 : Outport  Port=6
  wires:
  Extract Bits5/1 -> Out1/1
  Extract Bits4/1 -> Out2/1
  Extract Bits3/1 -> Out3/1
  Extract Bits2/1 -> Out4/1
  In1/1 -> bitnot/1
  Extract Bits1/1 -> Out5/1
  Extract Bits/1 -> Out6/1
  bitnot/1 -> Extract Bits1/1, Extract Bits2/1, Extract Bits3/1, Extract Bits5/1, Extract Bits4/1, Extract Bits/1

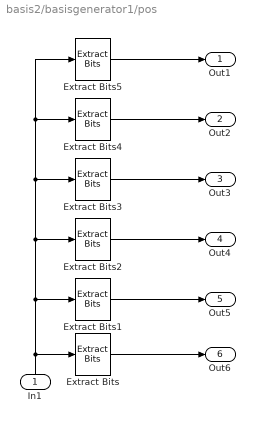
== system basis2/basisgenerator1/pos ==
  In1 : Inport  Orientation=up
  Extract Bits : simulink/Logic and Bit Operations/Extract Bits  SystemSampleTime=-1  bitsToExtract=Range of bits  numBits=8  bitIdxRange=[5 5]  outScalingMode=Treat bit field as an integer
  Extract Bits1 : simulink/Logic and Bit Operations/Extract Bits  SystemSampleTime=-1  bitsToExtract=Range of bits  numBits=8  bitIdxRange=[4 4]  outScalingMode=Treat bit field as an integer
  Extract Bits2 : simulink/Logic and Bit Operations/Extract Bits  SystemSampleTime=-1  bitsToExtract=Range of bits  numBits=8  bitIdxRange=[3 3]  outScalingMode=Treat bit field as an integer
  Extract Bits3 : simulink/Logic and Bit Operations/Extract Bits  SystemSampleTime=-1  bitsToExtract=Range of bits  numBits=8  bitIdxRange=[2 2]  outScalingMode=Treat bit field as an integer
  Extract Bits4 : simulink/Logic and Bit Operations/Extract Bits  SystemSampleTime=-1  bitsToExtract=Range of bits  numBits=8  bitIdxRange=[1 1]  outScalingMode=Treat bit field as an integer
  Extract Bits5 : simulink/Logic and Bit Operations/Extract Bits  SystemSampleTime=-1  bitsToExtract=Range of bits  numBits=8  bitIdxRange=[0 0]  outScalingMode=Treat bit field as an integer
  Out1 : Outport
  Out2 : Outport  Port=2
  Out3 : Outport  Port=3
  Out4 : Outport  Port=4
  Out5 : Outport  Port=5
  Out6 : Outport  Port=6
  wires:
  Extract Bits5/1 -> Out1/1
  Extract Bits4/1 -> Out2/1
  Extract Bits3/1 -> Out3/1
  Extract Bits2/1 -> Out4/1
  In1/1 -> Extract Bits1/1, Extract Bits2/1, Extract Bits3/1, Extract Bits5/1, Extract Bits4/1, Extract Bits/1
  Extract Bits1/1 -> Out5/1
  Extract Bits/1 -> Out6/1

== system basis2/corr/mux ==
  In1 : Inport
  In2 : Inport  Port=2
  C : MultiPortSwitch  Inputs=64  zeroidx=on
  Demux3 : Demux  Outputs=64
  Out1 : Outport
  wires:
  C/1 -> Out1/1
  In2/1 -> Demux3/1
  In1/1 -> C/1
  Demux3/1 -> C/2
  Demux3/2 -> C/3
  Demux3/3 -> C/4
  Demux3/4 -> C/5
  Demux3/5 -> C/6
  Demux3/6 -> C/7
  Demux3/7 -> C/8
  Demux3/8 -> C/9
  Demux3/9 -> C/10
  Demux3/10 -> C/11
  Demux3/11 -> C/12
  Demux3/12 -> C/13
  Demux3/13 -> C/14
  Demux3/15 -> C/16
  Demux3/16 -> C/17
  Demux3/17 -> C/18
  Demux3/18 -> C/19
  Demux3/19 -> C/20
  Demux3/20 -> C/21
  Demux3/21 -> C/22
  Demux3/22 -> C/23
  Demux3/23 -> C/24
  Demux3/24 -> C/25
  Demux3/25 -> C/26
  Demux3/26 -> C/27
  Demux3/27 -> C/28
  Demux3/28 -> C/29
  Demux3/29 -> C/30
  Demux3/30 -> C/31
  Demux3/31 -> C/32
  Demux3/32 -> C/33
  Demux3/33 -> C/34
  Demux3/34 -> C/35
  Demux3/35 -> C/36
  Demux3/36 -> C/37
  Demux3/37 -> C/38
  Demux3/38 -> C/39
  Demux3/39 -> C/40
  Demux3/40 -> C/41
  Demux3/41 -> C/42
  Demux3/42 -> C/43
  Demux3/43 -> C/44
  Demux3/44 -> C/45
  Demux3/45 -> C/46
  Demux3/46 -> C/47
  Demux3/47 -> C/48
  Demux3/48 -> C/49
  Demux3/49 -> C/50
  Demux3/50 -> C/51
  Demux3/51 -> C/52
  Demux3/52 -> C/53
  Demux3/53 -> C/54
  Demux3/54 -> C/55
  Demux3/55 -> C/56
  Demux3/56 -> C/57
  Demux3/57 -> C/58
  Demux3/58 -> C/59
  Demux3/59 -> C/60
  Demux3/60 -> C/61
  Demux3/61 -> C/62
  Demux3/62 -> C/63
  Demux3/63 -> C/64
  Demux3/64 -> C/65
  Demux3/14 -> C/15

== system basis2/corr1/mux ==
  In1 : Inport
  In2 : Inport  Port=2
  C : MultiPortSwitch  Inputs=64  zeroidx=on
  Demux3 : Demux  Outputs=64
  Out1 : Outport
  wires:
  C/1 -> Out1/1
  In2/1 -> Demux3/1
  In1/1 -> C/1
  Demux3/1 -> C/2
  Demux3/2 -> C/3
  Demux3/3 -> C/4
  Demux3/4 -> C/5
  Demux3/5 -> C/6
  Demux3/6 -> C/7
  Demux3/7 -> C/8
  Demux3/8 -> C/9
  Demux3/9 -> C/10
  Demux3/10 -> C/11
  Demux3/11 -> C/12
  Demux3/12 -> C/13
  Demux3/13 -> C/14
  Demux3/15 -> C/16
  Demux3/16 -> C/17
  Demux3/17 -> C/18
  Demux3/18 -> C/19
  Demux3/19 -> C/20
  Demux3/20 -> C/21
  Demux3/21 -> C/22
  Demux3/22 -> C/23
  Demux3/23 -> C/24
  Demux3/24 -> C/25
  Demux3/25 -> C/26
  Demux3/26 -> C/27
  Demux3/27 -> C/28
  Demux3/28 -> C/29
  Demux3/29 -> C/30
  Demux3/30 -> C/31
  Demux3/31 -> C/32
  Demux3/32 -> C/33
  Demux3/33 -> C/34
  Demux3/34 -> C/35
  Demux3/35 -> C/36
  Demux3/36 -> C/37
  Demux3/37 -> C/38
  Demux3/38 -> C/39
  Demux3/39 -> C/40
  Demux3/40 -> C/41
  Demux3/41 -> C/42
  Demux3/42 -> C/43
  Demux3/43 -> C/44
  Demux3/44 -> C/45
  Demux3/45 -> C/46
  Demux3/46 -> C/47
  Demux3/47 -> C/48
  Demux3/48 -> C/49
  Demux3/49 -> C/50
  Demux3/50 -> C/51
  Demux3/51 -> C/52
  Demux3/52 -> C/53
  Demux3/53 -> C/54
  Demux3/54 -> C/55
  Demux3/55 -> C/56
  Demux3/56 -> C/57
  Demux3/57 -> C/58
  Demux3/58 -> C/59
  Demux3/59 -> C/60
  Demux3/60 -> C/61
  Demux3/61 -> C/62
  Demux3/62 -> C/63
  Demux3/63 -> C/64
  Demux3/64 -> C/65
  Demux3/14 -> C/15

== system basis2/corr2/mux ==
  In1 : Inport
  In2 : Inport  Port=2
  C : MultiPortSwitch  Inputs=64  zeroidx=on
  Demux3 : Demux  Outputs=64
  Out1 : Outport
  wires:
  C/1 -> Out1/1
  In2/1 -> Demux3/1
  In1/1 -> C/1
  Demux3/1 -> C/2
  Demux3/2 -> C/3
  Demux3/3 -> C/4
  Demux3/4 -> C/5
  Demux3/5 -> C/6
  Demux3/6 -> C/7
  Demux3/7 -> C/8
  Demux3/8 -> C/9
  Demux3/9 -> C/10
  Demux3/10 -> C/11
  Demux3/11 -> C/12
  Demux3/12 -> C/13
  Demux3/13 -> C/14
  Demux3/15 -> C/16
  Demux3/16 -> C/17
  Demux3/17 -> C/18
  Demux3/18 -> C/19
  Demux3/19 -> C/20
  Demux3/20 -> C/21
  Demux3/21 -> C/22
  Demux3/22 -> C/23
  Demux3/23 -> C/24
  Demux3/24 -> C/25
  Demux3/25 -> C/26
  Demux3/26 -> C/27
  Demux3/27 -> C/28
  Demux3/28 -> C/29
  Demux3/29 -> C/30
  Demux3/30 -> C/31
  Demux3/31 -> C/32
  Demux3/32 -> C/33
  Demux3/33 -> C/34
  Demux3/34 -> C/35
  Demux3/35 -> C/36
  Demux3/36 -> C/37
  Demux3/37 -> C/38
  Demux3/38 -> C/39
  Demux3/39 -> C/40
  Demux3/40 -> C/41
  Demux3/41 -> C/42
  Demux3/42 -> C/43
  Demux3/43 -> C/44
  Demux3/44 -> C/45
  Demux3/45 -> C/46
  Demux3/46 -> C/47
  Demux3/47 -> C/48
  Demux3/48 -> C/49
  Demux3/49 -> C/50
  Demux3/50 -> C/51
  Demux3/51 -> C/52
  Demux3/52 -> C/53
  Demux3/53 -> C/54
  Demux3/54 -> C/55
  Demux3/55 -> C/56
  Demux3/56 -> C/57
  Demux3/57 -> C/58
  Demux3/58 -> C/59
  Demux3/59 -> C/60
  Demux3/60 -> C/61
  Demux3/61 -> C/62
  Demux3/62 -> C/63
  Demux3/63 -> C/64
  Demux3/64 -> C/65
  Demux3/14 -> C/15

== system basis2/pos/ws ==
  in0 : Inport
  in1 : Inport  Port=2
  in2 : Inport  Port=3
  Sum : Sum  Inputs=+++++++  SaturateOnIntegerOverflow=on  InputSameDT=on
  Out1 : Outport
  wires:
  Sum/1 -> Out1/1
  in0/1 -> Sum/1
  in1/1 -> Sum/2, Sum/3
  in2/1 -> Sum/4, Sum/5, Sum/6, Sum/7

== system basis2/basisgenerator/indgen0/ws ==
  In1 : Inport
  In2 : Inport  Port=2
  Sum : Sum  Inputs=+++  SaturateOnIntegerOverflow=on  InputSameDT=on
  Out1 : Outport
  wires:
  In1/1 -> Sum/2, Sum/1
  In2/1 -> Sum/3
  Sum/1 -> Out1/1

== system basis2/basisgenerator/indgen0/ws1 ==
  In1 : Inport
  In2 : Inport  Port=2
  Sum : Sum  Inputs=+++  SaturateOnIntegerOverflow=on  InputSameDT=on
  Out1 : Outport
  wires:
  In1/1 -> Sum/2, Sum/1
  In2/1 -> Sum/3
  Sum/1 -> Out1/1

== system basis2/basisgenerator/indgen0/ws2 ==
  In1 : Inport
  In2 : Inport  Port=2
  Sum : Sum  Inputs=+++  SaturateOnIntegerOverflow=on  InputSameDT=on
  Out1 : Outport
  wires:
  In1/1 -> Sum/2, Sum/1
  In2/1 -> Sum/3
  Sum/1 -> Out1/1

== system basis2/basisgenerator/indgen0/ws3 ==
  In1 : Inport
  In2 : Inport  Port=2
  Sum : Sum  Inputs=+++  SaturateOnIntegerOverflow=on  InputSameDT=on
  Out1 : Outport
  wires:
  In1/1 -> Sum/2, Sum/1
  In2/1 -> Sum/3
  Sum/1 -> Out1/1

== system basis2/basisgenerator/indgen1/ws ==
  In1 : Inport
  In2 : Inport  Port=2
  Sum : Sum  Inputs=+++  SaturateOnIntegerOverflow=on  InputSameDT=on
  Out1 : Outport
  wires:
  In1/1 -> Sum/2, Sum/1
  In2/1 -> Sum/3
  Sum/1 -> Out1/1

== system basis2/basisgenerator/indgen1/ws1 ==
  In1 : Inport
  In2 : Inport  Port=2
  Sum : Sum  Inputs=+++  SaturateOnIntegerOverflow=on  InputSameDT=on
  Out1 : Outport
  wires:
  In1/1 -> Sum/2, Sum/1
  In2/1 -> Sum/3
  Sum/1 -> Out1/1

== system basis2/basisgenerator/indgen1/ws2 ==
  In1 : Inport
  In2 : Inport  Port=2
  Sum : Sum  Inputs=+++  SaturateOnIntegerOverflow=on  InputSameDT=on
  Out1 : Outport
  wires:
  In1/1 -> Sum/2, Sum/1
  In2/1 -> Sum/3
  Sum/1 -> Out1/1

== system basis2/basisgenerator/indgen1/ws3 ==
  In1 : Inport
  In2 : Inport  Port=2
  Sum : Sum  Inputs=+++  SaturateOnIntegerOverflow=on  InputSameDT=on
  Out1 : Outport
  wires:
  In1/1 -> Sum/2, Sum/1
  In2/1 -> Sum/3
  Sum/1 -> Out1/1

== system basis2/basisgenerator/indgen2/ws ==
  In1 : Inport
  In2 : Inport  Port=2
  Sum : Sum  Inputs=+++  SaturateOnIntegerOverflow=on  InputSameDT=on
  Out1 : Outport
  wires:
  In1/1 -> Sum/2, Sum/1
  In2/1 -> Sum/3
  Sum/1 -> Out1/1

== system basis2/basisgenerator/indgen2/ws1 ==
  In1 : Inport
  In2 : Inport  Port=2
  Sum : Sum  Inputs=+++  SaturateOnIntegerOverflow=on  InputSameDT=on
  Out1 : Outport
  wires:
  In1/1 -> Sum/2, Sum/1
  In2/1 -> Sum/3
  Sum/1 -> Out1/1

== system basis2/basisgenerator/indgen2/ws2 ==
  In1 : Inport
  In2 : Inport  Port=2
  Sum : Sum  Inputs=+++  SaturateOnIntegerOverflow=on  InputSameDT=on
  Out1 : Outport
  wires:
  In1/1 -> Sum/2, Sum/1
  In2/1 -> Sum/3
  Sum/1 -> Out1/1

== system basis2/basisgenerator/indgen2/ws3 ==
  In1 : Inport
  In2 : Inport  Port=2
  Sum : Sum  Inputs=+++  SaturateOnIntegerOverflow=on  InputSameDT=on
  Out1 : Outport
  wires:
  In1/1 -> Sum/2, Sum/1
  In2/1 -> Sum/3
  Sum/1 -> Out1/1

== system basis2/basisgenerator1/indgen0/ws ==
  In1 : Inport
  In2 : Inport  Port=2
  Sum : Sum  Inputs=+++  SaturateOnIntegerOverflow=on  InputSameDT=on
  Out1 : Outport
  wires:
  In1/1 -> Sum/2, Sum/1
  In2/1 -> Sum/3
  Sum/1 -> Out1/1

== system basis2/basisgenerator1/indgen0/ws1 ==
  In1 : Inport
  In2 : Inport  Port=2
  Sum : Sum  Inputs=+++  SaturateOnIntegerOverflow=on  InputSameDT=on
  Out1 : Outport
  wires:
  In1/1 -> Sum/2, Sum/1
  In2/1 -> Sum/3
  Sum/1 -> Out1/1

== system basis2/basisgenerator1/indgen0/ws2 ==
  In1 : Inport
  In2 : Inport  Port=2
  Sum : Sum  Inputs=+++  SaturateOnIntegerOverflow=on  InputSameDT=on
  Out1 : Outport
  wires:
  In1/1 -> Sum/2, Sum/1
  In2/1 -> Sum/3
  Sum/1 -> Out1/1

== system basis2/basisgenerator1/indgen0/ws3 ==
  In1 : Inport
  In2 : Inport  Port=2
  Sum : Sum  Inputs=+++  SaturateOnIntegerOverflow=on  InputSameDT=on
  Out1 : Outport
  wires:
  In1/1 -> Sum/2, Sum/1
  In2/1 -> Sum/3
  Sum/1 -> Out1/1

== system basis2/basisgenerator1/indgen1/ws ==
  In1 : Inport
  In2 : Inport  Port=2
  Sum : Sum  Inputs=+++  SaturateOnIntegerOverflow=on  InputSameDT=on
  Out1 : Outport
  wires:
  In1/1 -> Sum/2, Sum/1
  In2/1 -> Sum/3
  Sum/1 -> Out1/1

== system basis2/basisgenerator1/indgen1/ws1 ==
  In1 : Inport
  In2 : Inport  Port=2
  Sum : Sum  Inputs=+++  SaturateOnIntegerOverflow=on  InputSameDT=on
  Out1 : Outport
  wires:
  In1/1 -> Sum/2, Sum/1
  In2/1 -> Sum/3
  Sum/1 -> Out1/1

== system basis2/basisgenerator1/indgen1/ws2 ==
  In1 : Inport
  In2 : Inport  Port=2
  Sum : Sum  Inputs=+++  SaturateOnIntegerOverflow=on  InputSameDT=on
  Out1 : Outport
  wires:
  In1/1 -> Sum/2, Sum/1
  In2/1 -> Sum/3
  Sum/1 -> Out1/1

== system basis2/basisgenerator1/indgen1/ws3 ==
  In1 : Inport
  In2 : Inport  Port=2
  Sum : Sum  Inputs=+++  SaturateOnIntegerOverflow=on  InputSameDT=on
  Out1 : Outport
  wires:
  In1/1 -> Sum/2, Sum/1
  In2/1 -> Sum/3
  Sum/1 -> Out1/1

== system basis2/basisgenerator1/indgen2/ws ==
  In1 : Inport
  In2 : Inport  Port=2
  Sum : Sum  Inputs=+++  SaturateOnIntegerOverflow=on  InputSameDT=on
  Out1 : Outport
  wires:
  In1/1 -> Sum/2, Sum/1
  In2/1 -> Sum/3
  Sum/1 -> Out1/1

== system basis2/basisgenerator1/indgen2/ws1 ==
  In1 : Inport
  In2 : Inport  Port=2
  Sum : Sum  Inputs=+++  SaturateOnIntegerOverflow=on  InputSameDT=on
  Out1 : Outport
  wires:
  In1/1 -> Sum/2, Sum/1
  In2/1 -> Sum/3
  Sum/1 -> Out1/1

== system basis2/basisgenerator1/indgen2/ws2 ==
  In1 : Inport
  In2 : Inport  Port=2
  Sum : Sum  Inputs=+++  SaturateOnIntegerOverflow=on  InputSameDT=on
  Out1 : Outport
  wires:
  In1/1 -> Sum/2, Sum/1
  In2/1 -> Sum/3
  Sum/1 -> Out1/1

== system basis2/basisgenerator1/indgen2/ws3 ==
  In1 : Inport
  In2 : Inport  Port=2
  Sum : Sum  Inputs=+++  SaturateOnIntegerOverflow=on  InputSameDT=on
  Out1 : Outport
  wires:
  In1/1 -> Sum/2, Sum/1
  In2/1 -> Sum/3
  Sum/1 -> Out1/1
